simulink model "EEControl"  (R2022a)
settings: Solver=VariableStepAuto  StartTime=0.0  StopTime=2  RelTol=1e-3
settings Model: Creator=nineb  LastModifiedBy=natha
settings DebuggingCC: UnconnectedInputMsg=warning  UnconnectedOutputMsg=warning  UnconnectedLineMsg=warning
settings RTWCC: DLArmComputeVersion=19.05

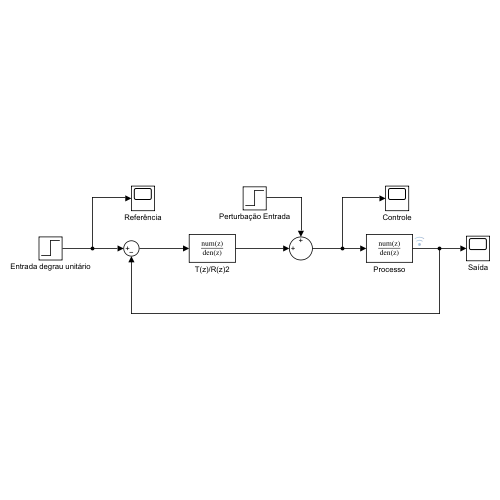
[thumbnail: Simulink's stored preview of the top-level diagram]
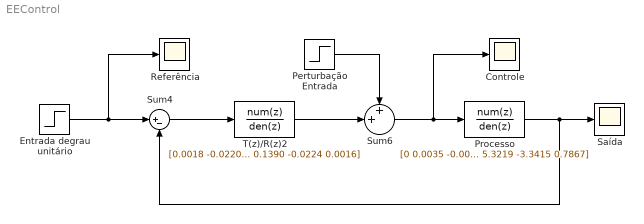
== system EEControl ==
  Controle : Scope
  Entrada degrau unitário : Step  Time=0  SampleTime=0.06
  Perturbação Entrada : Step  Time=15  After=0  SampleTime=0.06
  Processo : DiscreteTransferFcn  Numerator=[0 0.0035 -0.0033 -0.0031 0.0029]  Denominator=[1 -3.7672 5.3219 -3.3415 0.7867]  SampleTime=0.06
  Referência : Scope
  Saída : Scope
  Sum4 : Sum  Inputs=|+-
  Sum6 : Sum  Inputs=++|
  T(z)/R(z)2 : DiscreteTransferFcn  Numerator=[0.0018 -0.0220 0.1236 -0.4166 0.9247 -1.3852 1.3286 -0.5689 -0.4587 1.0758 -1.0325 0.6267 -0.2556 0.0686 -0.0110 8.0415e-04]  Denominator=[0.0035 -0.0433 0.2443 -0.8254 1.8379 -2.7633 2.6639 -1.1575 -0.8983 2.1455 -2.0708 1.2619 -0.5166 0.1390 -0.0224 0.0016]  SampleTime=0.06
  wires:
  Processo/1 -> Sum4/2, Saída/1
  Perturbação Entrada/1 -> Sum6/1
  Entrada degrau unitário/1 -> Referência/1, Sum4/1
  Sum6/1 -> Processo/1, Controle/1
  T(z)/R(z)2/1 -> Sum6/2
  Sum4/1 -> T(z)/R(z)2/1
